simulink model "test_blow"  (R2013a)
settings: Solver=ode45  StartTime=0.0  StopTime=100.0  RelTol=1e-3
undefined symbols (not defined in the file): dfilt, eval_time_samples, magnitude, n_pow_thres, n_sat_thres, pow_thresh_high, pow_thresh_low, sat_thresh
libraries: dsparch4 x2, etargetslib x1, instrumentlib x1
settings Model: SimulationMode=accelerator  Creator=leonardo  LastModifiedBy=Leonardo

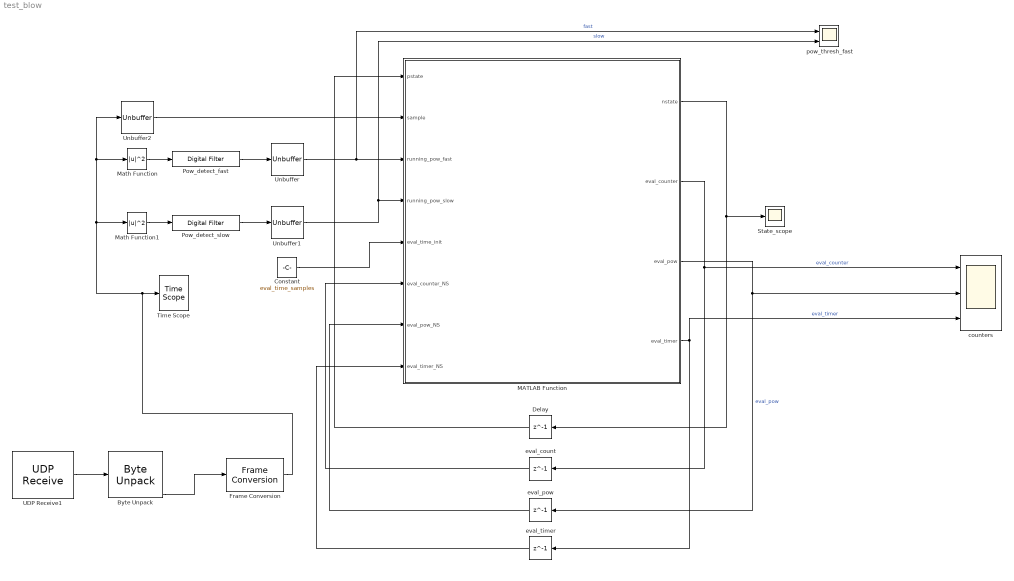
== system test_blow ==
  Byte Unpack : etargetslib/Byte Unpack  dimensions={[1],[1],[1 2],[1 2],[1],[1],[(2080-32)/4 1]}  datatypes={'int32','int32','uint32','uint32','int32','int32','single'}  byteAlign=1
  Constant : Constant  Value=eval_time_samples  SampleTime=1/44100
  Delay : Delay  DelayLength=1  InitialCondition=1
  Frame Conversion : FrameConversion
  MATLAB Function : MATLAB Function  TreatAsAtomicUnit=on
  Math Function : Math  Operator=magnitude^2  SaturateOnIntegerOverflow=on
  Math Function1 : Math  Operator=magnitude^2  SaturateOnIntegerOverflow=on
  Pow_detect_fast : dsparch4/Digital Filter  TypePopup=FIR (all zeros)  IIRFiltStruct=Direct form II transposed  AllPoleFiltStruct=Direct form  FIRFiltStruct=Direct form  CoeffSource=Specify via dialog  NumCoeffs=bb_fast  DenCoeffs=[1 0.1]  BiQuadCoeffs=[1 0.3 0.4 1 0.1 0.2]  LatticeCoeffs=[0.2 0.4]  denIgnore=on  FiltPerSampPopup=One filter per frame  IC=0  ICnum=0  ICden=0  roundingMode=Floor  overflowMode=off  ScaleValues=1  scaleValueFracLength=14  stageInFracLength=15  stageOutFracLength=15  FilterSource=Specify via dialog  dfiltObjectName=dfilt.dffir([1 2 1])  InputProcessing=Columns as channels (frame based)
  Pow_detect_slow : dsparch4/Digital Filter  TypePopup=FIR (all zeros)  IIRFiltStruct=Direct form II transposed  AllPoleFiltStruct=Direct form  FIRFiltStruct=Direct form  CoeffSource=Specify via dialog  NumCoeffs=bb_slow  DenCoeffs=[1 0.1]  BiQuadCoeffs=[1 0.3 0.4 1 0.1 0.2]  LatticeCoeffs=[0.2 0.4]  denIgnore=on  FiltPerSampPopup=One filter per frame  IC=0  ICnum=0  ICden=0  roundingMode=Floor  overflowMode=off  ScaleValues=1  scaleValueFracLength=14  stageInFracLength=15  stageOutFracLength=15  FilterSource=Specify via dialog  dfiltObjectName=dfilt.dffir([1 2 1])  InputProcessing=Columns as channels (frame based)
  State_scope : Scope
      settings: YMin=1.9  YMax=2.1
  Time Scope : TimeScope  DefaultConfigurationName=spbscopes.TimeScopeBlockCfg
      settings: CopyFcn=scopeextensions.ScopeBlock.callback(gcbh, 'onBlockCopy', gcbh);  DeleteFcn=scopeextensions.ScopeBlock.callback(gcbh, 'onBlockDelete');  PreSaveFcn=scopeextensions.ScopeBlock.callback(gcbh, 'onModelSave');  NameChangeFcn=scopeextensions.ScopeBlock.callback(gcbh, 'onBlockRename');  CloseFcn=scopeextensions.ScopeBlock.callback(gcbh, 'onBlockClose');  PreDeleteFcn=scopeextensions.ScopeBlock.callback(gcbh, 'onBlockPreDelete');
  UDP Receive1 : instrumentlib/UDP Receive  Host=192.168.1.14  Port=61538  LocalPort=50000  DataSize="[1  2080]"  EnableBlockingMode=on  Timeout=10  SampleTime=512/44100  DataType=uint8  ByteOrder=BigEndian
  Unbuffer : Unbuffer  SampleBasedProcessing=Same as frame based
  Unbuffer1 : Unbuffer  SampleBasedProcessing=Same as frame based
  Unbuffer2 : Unbuffer  SampleBasedProcessing=Same as frame based
  counters : Scope  NumInputPorts=3
      settings: YMin=33.25~-1~2052.95  YMax=36.75~1~2269.05  SaveName=ScopeData2
  eval_count : Delay  DelayLength=1  InitialCondition=0
  eval_pow : Delay  DelayLength=1  InitialCondition=0
  eval_timer : Delay  DelayLength=1  InitialCondition=0
  pow_thresh_fast : Scope  NumInputPorts=2
      settings: YMin=1.9~-5  YMax=2.1~5
  wires:
  MATLAB Function/1(nstate) -> State_scope/1, Delay/1
  Delay/1 -> MATLAB Function/1(pstate)
  Pow_detect_fast/1 -> Unbuffer/1
  Pow_detect_slow/1 -> Unbuffer1/1
  Constant/1 -> MATLAB Function/5(eval_time_init)
  Math Function/1 -> Pow_detect_fast/1
  Math Function1/1 -> Pow_detect_slow/1
  Frame Conversion/1 -> Unbuffer2/1, Math Function/1, Math Function1/1, Time Scope/1
  Unbuffer/1 -> pow_thresh_fast/1, MATLAB Function/3(running_pow_fast)  "fast"
  Unbuffer1/1 -> pow_thresh_fast/2, MATLAB Function/4(running_pow_slow)  "slow"
  Unbuffer2/1 -> MATLAB Function/2(sample)
  MATLAB Function/2(eval_counter) -> eval_count/1, counters/1  "eval_counter"
  eval_count/1 -> MATLAB Function/6(eval_counter_NS)
  MATLAB Function/4(eval_timer) -> eval_timer/1, counters/3  "eval_timer"
  MATLAB Function/3(eval_pow) -> counters/2, eval_pow/1  "eval_pow"
  eval_pow/1 -> MATLAB Function/7(eval_pow_NS)
  eval_timer/1 -> MATLAB Function/8(eval_timer_NS)
  UDP Receive1/1 -> Byte Unpack/1
  Byte Unpack/7 -> Frame Conversion/1

== matlab function test_blow/MATLAB Function ==
  data: pstate input; nstate output; sample input; running_pow_fast input; running_pow_slow input; pow_thresh_high parameter; pow_thresh_low parameter; sat_thresh parameter; n_sat_thres parameter; n_pow_thres parameter; eval_time_init input; eval_counter_NS input; eval_pow_NS input; eval_timer_NS input; eval_counter output; eval_pow output; eval_timer output
function  [nstate,eval_counter,eval_pow,eval_timer] =saturation_detector(pstate,sample,running_pow_fast,running_pow_slow,pow_thresh_high,pow_thresh_low,sat_thresh,n_sat_thres,n_pow_thres,eval_time_init,...
    eval_counter_NS,eval_pow_NS,eval_timer_NS)
%#codegen

% persistent eval_counter_NS;
% persistent eval_pow_NS;
% persistent eval_timer_NS;
% persistent frame_n_latch;
% persistent win_counter;

% State_waiting.Name='waiting'; %1
State_waiting=1;
% State_waiting.Id  = 1;
% State_evaluation.Name='evaluation';%2
% State_evaluation.Id  = 2;
State_evaluation=2;
% State_trackin.Name='trackin';%3
% State_trackin.Id  = 3;
State_trackin=3;


% if isempty(eval_counter_NS)
%     eval_counter_NS=0;
% end
% 
% if isempty(eval_timer_NS)
%     eval_timer_NS=0;
% end
% 
% if isempty(eval_pow_NS)
%     eval_pow_NS=0;
% end

% if isempty(win_counter)
%     win_counter=0;
% end

% running_pow_len = frame_n_latch*frame_len+sample_idx;

% switch pstate.Idpow_acc

% for sample_idx=1:length(frame)

    if pstate==State_trackin
        

        if running_pow_slow<=pow_thresh_low
            eval_pow=eval_pow_NS+1;
        else
            eval_pow=eval_pow_NS;
        end

       if eval_pow>n_pow_thres
            nstate=State_waiting;
        else
             nstate=pstate;
       end
        
       eval_counter=eval_counter_NS;
       eval_timer=eval_timer_NS;
        
         
%         if sample_idx==frame_len
%             frame_n_latch=frame_n_latch+1;
%         end
    
    elseif pstate==State_evaluation
        eval_timer=eval_timer_NS-1;

       
        if abs(sample)>sat_thresh
            eval_counter=eval_counter_NS+1;
         else
             eval_counter=eval_counter_NS;
        end
        if running_pow_fast>=pow_thresh_high
            eval_pow=eval_pow_NS+1;
        else
            eval_pow=eval_pow_NS;
        end
%         running_pow_fast=pow_acc/win_counter;

        if eval_counter>n_sat_thres && eval_timer>=0 && eval_pow>=n_pow_thres
            
            nstate=State_trackin;
            eval_pow=0;
%              running_pow_fast=(running_pow_fast*(win_counter-1)+frame)/win_counter;
%             running_pow_fast=running_pow_fast/sample_idx;

        elseif eval_timer==0

            nstate=State_waiting;
            
        else
            nstate=State_evaluation;
        end
        
%         if sample_idx==frame_len
%             frame_n_latch=frame_n_latch+1;
%         end
    
    
    elseif pstate==State_waiting
%         frame_n_latch=0;
        
        if sample>sat_thresh

            eval_timer=eval_time_init;
            eval_counter=0;
            eval_pow= 0;
%              win_counter=0;
%             pow_acc=0;
            nstate=State_evaluation;
        else
            eval_timer=eval_timer_NS;
             eval_counter= eval_counter_NS;
             eval_pow=eval_pow_NS;
            nstate=State_waiting;

        end
        
    else
        
%         pstate
        error('State Unknown');
% end
    
    
    end
    
%     eval_counter=eval_counter_NS;
% eval_pow=eval_pow_NS;
% eval_timer=eval_timer_NS;
    
end


% end
